simulink model "TWAICE_Cell_Model_Farasis_P75_75Ah_v8_1_3"  (R2017b)
settings: Solver=ode3  StartTime=t_start  StopTime=t_end  FixedStep=Ts  RelTol=1e-3
InitFcn:
  | m = Simulink.Mask.get(strcat(model,'/Virtual Battery Tester'));
  | cycler_selection_sel = m.getParameter('cycler_selection');
  | ts_data_repeat_tickbox_sel = m.getParameter('ts_data_repeat_tickbox');
  | if strcmp(cycler_selection_sel.Value, 'Cycle Generator')
  |      t_end = 60*60*24*365*8;
  | elseif strcmp(cycler_selection_sel.Value, 'Timeseries Data')
  |      if strcmp(ts_data_repeat_tickbox_sel.Value, 'off')
  |           t_end = Data.Time(end);
  |      elseif strcmp(ts_data_repeat_tickbox_sel.Value, 'on')
  |            t_end = 60*60*24*365*8;
  |      end
  | end
StartFcn:
  | m = Simulink.Mask.get(strcat(model,'/Virtual Battery Tester'));
  | cycler_selection_sel = m.getParameter('cycler_selection');
  | ts_data_repeat_tickbox_sel = m.getParameter('ts_data_repeat_tickbox');
  | if strcmp(cycler_selection_sel.Value, 'Cycle Generator')
  |      t_end = 60*60*24*365*8;
  | elseif strcmp(cycler_selection_sel.Value, 'Timeseries Data')
  |      if strcmp(ts_data_repeat_tickbox_sel.Value, 'off')
  |           t_end = Data.Time(end);
  |      elseif strcmp(ts_data_repeat_tickbox_sel.Value, 'on')
  |            t_end = 60*60*24*365*8;
  |      end
  | end
model workspace (MAT data in the model file):
  SOC_init = 1
values from neighbouring files (symbols this model uses):
  act = 1    [RunMe_TWAICE_Cell_Model_Farasis_P75_75Ah_v8_1_3.m]
  I_chlim = []    [RunMe_TWAICE_Cell_Model_Farasis_P75_75Ah_v8_1_3.m]
  I_dislim = []    [RunMe_TWAICE_Cell_Model_Farasis_P75_75Ah_v8_1_3.m]
  lic_no = fin_convert(Prod_lic)    [RunMe_TWAICE_Cell_Model_Farasis_P75_75Ah_v8_1_3.m]
  model = 'TWAICE_Cell_Model_Farasis_P75_75Ah_v8_1_3'    [RunMe_TWAICE_Cell_Model_Farasis_P75_75Ah_v8_1_3.m]
  soc_chlim = chargelim.Var2(inx_soc:end)'    [RunMe_TWAICE_Cell_Model_Farasis_P75_75Ah_v8_1_3.m]
  soc_dislim = dischargelim.Var2(inx_soc:end)'    [RunMe_TWAICE_Cell_Model_Farasis_P75_75Ah_v8_1_3.m]
  T_chlim = []    [RunMe_TWAICE_Cell_Model_Farasis_P75_75Ah_v8_1_3.m]
  T_dislim = []    [RunMe_TWAICE_Cell_Model_Farasis_P75_75Ah_v8_1_3.m]
  Ts = 1    [RunMe_TWAICE_Cell_Model_Farasis_P75_75Ah_v8_1_3.m]
undefined symbols (not defined in the file or in its folder): Data, T_init
libraries: simulink x3
(part 2 of 2)

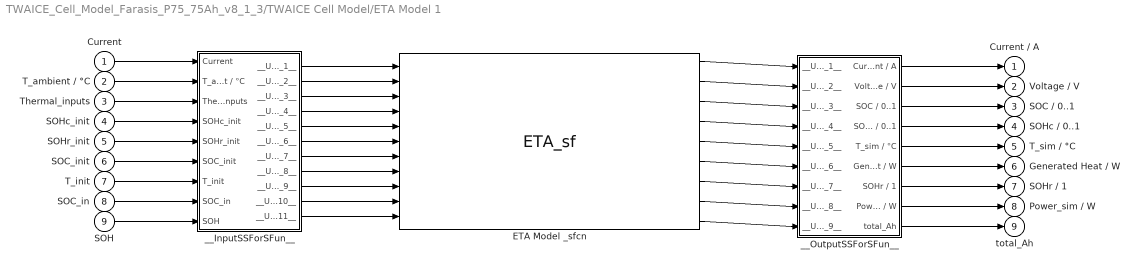
== system TWAICE_Cell_Model_Farasis_P75_75Ah_v8_1_3/TWAICE Cell Model/ETA Model 1 ==
  "Current " : Inport  OutDataTypeStr=double  PortDimensions=1
  T_ambient / °C : Inport  Port=2  OutDataTypeStr=double  PortDimensions=1
  Thermal_inputs : Inport  Port=3
  SOHc_init : Inport  Port=4
  SOHr_init : Inport  Port=5
  SOC_init : Inport  Port=6
  T_init : Inport  Port=7
  SOC_in : Inport  Port=8
  SOH : Inport  Port=9
  ETA Model _sfcn : S-Function  FunctionName=ETA_sf  Parameters=sfcnParam1, sfcnParam2, sfcnParam3  SFunctionModules=""  SFunctionDeploymentMode=off  EnableBusSupport=off  SFcnStateName=DWORK0  mask{rtw_sf_name=ETA_sf, showVar=off, sfcnParam1=sfcnParam1, sfcnParam2=sfcnParam2, sfcnParam3=sfcnParam3}
      mask prompts: rtw_sf_name "Simulink:masks:GenSFuncName_MP"; showVar "Simulink:masks:GenSFuncShowModuleList_MP"; sfcnParam1 "Ts:"; sfcnParam2 "act:"; sfcnParam3 "lic_no:"
      mask help: Simulink:masks:GenSFuncDesc_MD
      mask init:
      | displist = '';
      | if ~strcmp(get_param(gcb, 'FunctionName'), rtw_sf_name);
      |   set_param(gcb, 'FunctionName', rtw_sf_name);
      | end
      | % Check if we are generating code
      | rtw_mode = false;
      | if strcmpi(get_param(bdroot(gcb),'SimulationStatus'),'Initializing')
      | 	rtw_mode = strcmpi(get_param(bdroot(gcb),'BuildingRTWCode'),'on') && ...
      | 		~strcmpi(get_param(bdroot(gcb),'TargetStyle'),'SimulationTarget');
      | end
      | if showVar || rtw_mode
      | 	if exist('rtwsfunc') == 2 | exist('rtwsfunc') == 6
      | 		tmplist = rtwsfunc(rtw_sf_name,gcb);
      | 		tmplist = DAStudio.message('Simulink:masks:GenSFuncListOfModules_IC', tmplist);
      | 	elseif showVar
      | 		tmplist1 = DAStudio.message('Simulink:masks:GenSFuncListOfModules_IC', '');
      |         tmplist2 = DAStudio.message('Simulink:masks:GenSFuncNotLicensed_IC');
      |         tmplist = [tmplist1 tmplist2];
      |  	end
      | end
      | if showVar
      |   displist = tmplist;
      | end
      settings: SFcnIsStateOwnerBlock=on
      settings: CopyFcn=|
      | if ~strcmp(get_param(gcb,'Linkstatus'),'none') && ...
      | ~strcmp(get_param(gcb,'Linkstatus'),'implicit')
      |   set_param(gcb,'LinkStatus','none');
      | end
      mask Help: eval('feval(''rtwprivate'',''rtwhelpview'',''rtw_sfcn_block'')');
      mask Display:
      | port_label('input',1,'Current ');
      | port_label('input',2,'T_ambient / °C');
      | port_label('input',3,'htc_in');
      | port_label('input',4,'Pcool_in');
      | port_label('input',5,'SOHc_init');
      | port_label('input',6,'SOHr_init');
      | port_label('input',7,'SOC_init');
      | port_label('input',8,'T_init');
      | port_label('input',9,'SOC_in');
      | port_label('input',10,'SOHc');
      | port_label('input',11,'SOHr');
      | port_label('output',1,'Current / A');
      | port_label('output',2,'Voltage / V');
      | port_label('output',3,'SOC / 0..1');
      | port_label('output',4,'SOHc / 0..1');
      | port_label('output',5,'T_sim / °C');
      | port_label('output',6,'Generated Heat / W');
      | port_label('output',7,'SOHr / 1');
      | port_label('output',8,'Power_sim / W');
      | port_label('output',9,'total_Ah');
  __InputSSForSFun__ : Subsystem
  __OutputSSForSFun__ : Subsystem
  Current / A : Outport  OutDataTypeStr=double  PortDimensions=1  VectorParamsAs1DForOutWhenUnconnected=on
  Voltage / V : Outport  Port=2  OutDataTypeStr=double  PortDimensions=1  VectorParamsAs1DForOutWhenUnconnected=on
  SOC / 0..1 : Outport  Port=3  OutDataTypeStr=double  PortDimensions=1  VectorParamsAs1DForOutWhenUnconnected=on
  SOHc / 0..1 : Outport  Port=4  OutDataTypeStr=double  PortDimensions=1  VectorParamsAs1DForOutWhenUnconnected=on
  T_sim / °C : Outport  Port=5  OutDataTypeStr=double  PortDimensions=1  VectorParamsAs1DForOutWhenUnconnected=on
  Generated Heat / W : Outport  Port=6  OutDataTypeStr=double  PortDimensions=1  VectorParamsAs1DForOutWhenUnconnected=on
  SOHr / 1 : Outport  Port=7  OutDataTypeStr=double  PortDimensions=1  VectorParamsAs1DForOutWhenUnconnected=on
  Power_sim / W : Outport  Port=8  OutDataTypeStr=double  PortDimensions=1  VectorParamsAs1DForOutWhenUnconnected=on
  total_Ah : Outport  Port=9  VectorParamsAs1DForOutWhenUnconnected=on
  wires:
  "Current "/1 -> __InputSSForSFun__/1("Current ")
  T_ambient / °C/1 -> __InputSSForSFun__/2(T_ambient / °C)
  Thermal_inputs/1 -> __InputSSForSFun__/3(Thermal_inputs)
  SOHc_init/1 -> __InputSSForSFun__/4(SOHc_init)
  SOHr_init/1 -> __InputSSForSFun__/5(SOHr_init)
  SOC_init/1 -> __InputSSForSFun__/6(SOC_init)
  T_init/1 -> __InputSSForSFun__/7(T_init)
  SOC_in/1 -> __InputSSForSFun__/8(SOC_in)
  SOH/1 -> __InputSSForSFun__/9(SOH)
  __InputSSForSFun__/1(__UniqueOutportName__1__) -> ETA Model _sfcn/1
  __InputSSForSFun__/2(__UniqueOutportName__2__) -> ETA Model _sfcn/2
  __InputSSForSFun__/3(__UniqueOutportName__3__) -> ETA Model _sfcn/3
  __InputSSForSFun__/4(__UniqueOutportName__4__) -> ETA Model _sfcn/4
  __InputSSForSFun__/5(__UniqueOutportName__5__) -> ETA Model _sfcn/5
  __InputSSForSFun__/6(__UniqueOutportName__6__) -> ETA Model _sfcn/6
  __InputSSForSFun__/7(__UniqueOutportName__7__) -> ETA Model _sfcn/7
  __InputSSForSFun__/8(__UniqueOutportName__8__) -> ETA Model _sfcn/8
  __InputSSForSFun__/9(__UniqueOutportName__9__) -> ETA Model _sfcn/9
  __InputSSForSFun__/10(__UniqueOutportName__10__) -> ETA Model _sfcn/10
  __InputSSForSFun__/11(__UniqueOutportName__11__) -> ETA Model _sfcn/11
  ETA Model _sfcn/1 -> __OutputSSForSFun__/1(__UniqueInportName__1__)
  ETA Model _sfcn/2 -> __OutputSSForSFun__/2(__UniqueInportName__2__)
  ETA Model _sfcn/3 -> __OutputSSForSFun__/3(__UniqueInportName__3__)
  ETA Model _sfcn/4 -> __OutputSSForSFun__/4(__UniqueInportName__4__)
  ETA Model _sfcn/5 -> __OutputSSForSFun__/5(__UniqueInportName__5__)
  ETA Model _sfcn/6 -> __OutputSSForSFun__/6(__UniqueInportName__6__)
  ETA Model _sfcn/7 -> __OutputSSForSFun__/7(__UniqueInportName__7__)
  ETA Model _sfcn/8 -> __OutputSSForSFun__/8(__UniqueInportName__8__)
  ETA Model _sfcn/9 -> __OutputSSForSFun__/9(__UniqueInportName__9__)
  __OutputSSForSFun__/1(Current / A) -> Current / A/1
  __OutputSSForSFun__/2(Voltage / V) -> Voltage / V/1
  __OutputSSForSFun__/3(SOC / 0..1) -> SOC / 0..1/1
  __OutputSSForSFun__/4(SOHc / 0..1) -> SOHc / 0..1/1
  __OutputSSForSFun__/5(T_sim / °C) -> T_sim / °C/1
  __OutputSSForSFun__/6(Generated Heat / W) -> Generated Heat / W/1
  __OutputSSForSFun__/7(SOHr / 1) -> SOHr / 1/1
  __OutputSSForSFun__/8(Power_sim / W) -> Power_sim / W/1
  __OutputSSForSFun__/9(total_Ah) -> total_Ah/1

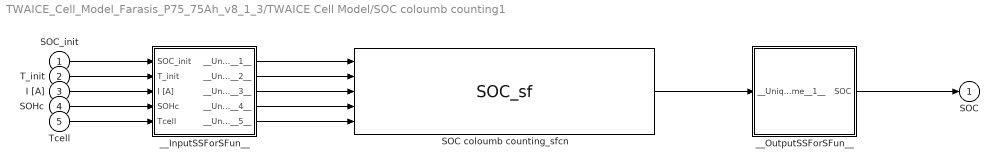
== system TWAICE_Cell_Model_Farasis_P75_75Ah_v8_1_3/TWAICE Cell Model/SOC coloumb counting1 ==
  SOC_init : Inport
  T_init : Inport  Port=2
  I [A] : Inport  Port=3
  SOHc : Inport  Port=4
  Tcell : Inport  Port=5
  SOC coloumb counting_sfcn : S-Function  FunctionName=SOC_sf  Parameters=sfcnParam1  SFunctionModules=""  SFunctionDeploymentMode=off  EnableBusSupport=off  SFcnStateName=DWORK0  mask{rtw_sf_name=SOC_sf, showVar=off, sfcnParam1=sfcnParam1}
      mask prompts: rtw_sf_name "Simulink:masks:GenSFuncName_MP"; showVar "Simulink:masks:GenSFuncShowModuleList_MP"; sfcnParam1 "Ts:"
      mask help: Simulink:masks:GenSFuncDesc_MD
      mask init: same as TWAICE_Cell_Model_Farasis_P75_75Ah_v8_1_3/TWAICE Cell Model/ETA Model 1/ETA Model _sfcn
      settings: SFcnIsStateOwnerBlock=on
      settings: CopyFcn=|
      | if ~strcmp(get_param(gcb,'Linkstatus'),'none') && ...
      | ~strcmp(get_param(gcb,'Linkstatus'),'implicit')
      |   set_param(gcb,'LinkStatus','none');
      | end
      mask Help: eval('feval(''rtwprivate'',''rtwhelpview'',''rtw_sfcn_block'')');
      mask Display:
      | port_label('input',1,'SOC_init');
      | port_label('input',2,'T_init');
      | port_label('input',3,'I [A]');
      | port_label('input',4,'SOHc');
      | port_label('input',5,'Tcell');
      | port_label('output',1,'SOC');
  __InputSSForSFun__ : Subsystem
  __OutputSSForSFun__ : Subsystem
  SOC : Outport
  wires:
  SOC_init/1 -> __InputSSForSFun__/1(SOC_init)
  T_init/1 -> __InputSSForSFun__/2(T_init)
  I [A]/1 -> __InputSSForSFun__/3(I [A])
  SOHc/1 -> __InputSSForSFun__/4(SOHc)
  Tcell/1 -> __InputSSForSFun__/5(Tcell)
  __InputSSForSFun__/1(__UniqueOutportName__1__) -> SOC coloumb counting_sfcn/1
  __InputSSForSFun__/2(__UniqueOutportName__2__) -> SOC coloumb counting_sfcn/2
  __InputSSForSFun__/3(__UniqueOutportName__3__) -> SOC coloumb counting_sfcn/3
  __InputSSForSFun__/4(__UniqueOutportName__4__) -> SOC coloumb counting_sfcn/4
  __InputSSForSFun__/5(__UniqueOutportName__5__) -> SOC coloumb counting_sfcn/5
  SOC coloumb counting_sfcn/1 -> __OutputSSForSFun__/1(__UniqueInportName__1__)
  __OutputSSForSFun__/1(SOC) -> SOC/1

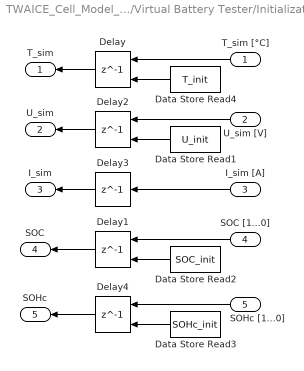
== system TWAICE_Cell_Model_Farasis_P75_75Ah_v8_1_3/Virtual Battery Tester/Initialization ==
  T_sim [°C] : Inport
  U_sim [V] : Inport  Port=2
  I_sim [A] : Inport  Port=3
  SOC [1...0] : Inport  Port=4
  SOHc [1...0] : Inport  Port=5
  Data Store Read1 : DataStoreRead  DataStoreName=U_init
  Data Store Read2 : DataStoreRead  DataStoreName=SOC_init
  Data Store Read3 : DataStoreRead  DataStoreName=SOHc_init
  Data Store Read4 : DataStoreRead  DataStoreName=T_init
  Delay : Delay  DelayLength=1  InitialConditionSource=Input port  InitialCondition=T_init
      settings: InputPortMap=u0,p4
  Delay1 : Delay  DelayLength=1  InitialConditionSource=Input port  InitialCondition=SOC_init
      settings: InputPortMap=u0,p4
  Delay2 : Delay  DelayLength=1  InitialConditionSource=Input port  InitialCondition=3.6
      settings: InputPortMap=u0,p4
  Delay3 : Delay  DelayLength=1  InitialCondition=0
  Delay4 : Delay  DelayLength=1  InitialConditionSource=Input port  InitialCondition=SOC_init
      settings: InputPortMap=u0,p4
  T_sim : Outport  VectorParamsAs1DForOutWhenUnconnected=on
  U_sim : Outport  Port=2  VectorParamsAs1DForOutWhenUnconnected=on
  I_sim : Outport  Port=3  VectorParamsAs1DForOutWhenUnconnected=on
  SOC : Outport  Port=4  VectorParamsAs1DForOutWhenUnconnected=on
  SOHc : Outport  Port=5  VectorParamsAs1DForOutWhenUnconnected=on
  wires:
  T_sim [°C]/1 -> Delay/1
  Delay1/1 -> SOC/1
  Delay2/1 -> U_sim/1
  SOC [1...0]/1 -> Delay1/1
  Delay/1 -> T_sim/1
  I_sim [A]/1 -> Delay3/1
  Delay3/1 -> I_sim/1
  SOHc [1...0]/1 -> Delay4/1
  U_sim [V]/1 -> Delay2/1
  Data Store Read2/1 -> Delay1/2
  Delay4/1 -> SOHc/1
  Data Store Read3/1 -> Delay4/2
  Data Store Read4/1 -> Delay/2
  Data Store Read1/1 -> Delay2/2

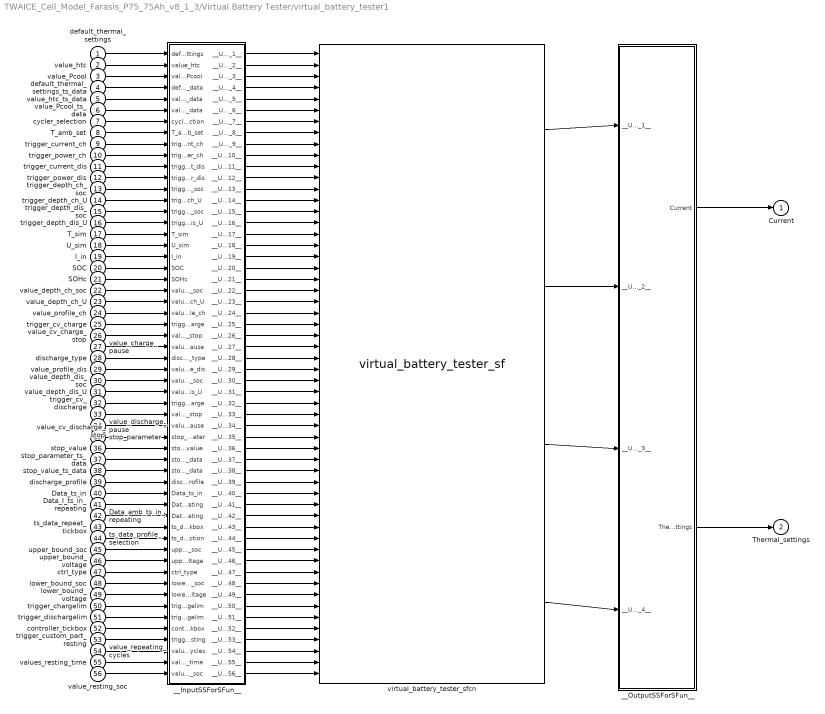
== system TWAICE_Cell_Model_Farasis_P75_75Ah_v8_1_3/Virtual Battery Tester/virtual_battery_tester1 ==
  default_thermal_settings : Inport
  value_htc : Inport  Port=2
  value_Pcool : Inport  Port=3
  default_thermal_settings_ts_data : Inport  Port=4
  value_htc_ts_data : Inport  Port=5
  value_Pcool_ts_data : Inport  Port=6
  cycler_selection : Inport  Port=7
  T_amb_set : Inport  Port=8
  trigger_current_ch : Inport  Port=9
  trigger_power_ch : Inport  Port=10
  trigger_current_dis : Inport  Port=11
  trigger_power_dis : Inport  Port=12
  trigger_depth_ch_soc : Inport  Port=13
  trigger_depth_ch_U : Inport  Port=14
  trigger_depth_dis_soc : Inport  Port=15
  trigger_depth_dis_U : Inport  Port=16
  T_sim : Inport  Port=17
  U_sim : Inport  Port=18
  I_in : Inport  Port=19
  SOC : Inport  Port=20
  SOHc : Inport  Port=21
  value_depth_ch_soc : Inport  Port=22
  value_depth_ch_U : Inport  Port=23
  value_profile_ch : Inport  Port=24
  trigger_cv_charge : Inport  Port=25
  value_cv_charge_stop : Inport  Port=26
  value_charge_pause : Inport  Port=27
  discharge_type : Inport  Port=28
  value_profile_dis : Inport  Port=29
  value_depth_dis_soc : Inport  Port=30
  value_depth_dis_U : Inport  Port=31
  trigger_cv_discharge : Inport  Port=32
  value_cv_discharge_stop : Inport  Port=33
  value_discharge_pause : Inport  Port=34
  stop_parameter : Inport  Port=35
  stop_value : Inport  Port=36
  stop_parameter_ts_data : Inport  Port=37
  stop_value_ts_data : Inport  Port=38
  discharge_profile : Inport  Port=39
  Data_ts_in : Inport  Port=40
  Data_I_ts_in_repeating : Inport  Port=41
  Data_amb_ts_in_repeating : Inport  Port=42
  ts_data_repeat_tickbox : Inport  Port=43
  ts_data_profile_selection : Inport  Port=44
  upper_bound_soc : Inport  Port=45
  upper_bound_voltage : Inport  Port=46
  ctrl_type : Inport  Port=47
  lower_bound_soc : Inport  Port=48
  lower_bound_voltage : Inport  Port=49
  trigger_chargelim : Inport  Port=50
  trigger_dischargelim : Inport  Port=51
  controller_tickbox : Inport  Port=52
  trigger_custom_part_resting : Inport  Port=53
  value_repeating_cycles : Inport  Port=54
  values_resting_time : Inport  Port=55
  value_resting_soc : Inport  Port=56
  __InputSSForSFun__ : Subsystem
  __OutputSSForSFun__ : Subsystem
  virtual_battery_tester_sfcn : S-Function  FunctionName=virtual_battery_tester_sf  Parameters=sfcnParam1, sfcnParam2, sfcnParam3, sfcnParam4, sfcnParam5, sfcnParam6, sfcnParam7, sfcnParam8  SFunctionModules=""  SFunctionDeploymentMode=off  EnableBusSupport=off  SFcnStateName=DWORK0  mask{rtw_sf_name=virtual_battery_tester_sf, showVar=off, sfcnParam1=sfcnParam1, sfcnParam2=sfcnParam2, sfcnParam3=sfcnParam3, sfcnParam4=sfcnParam4, sfcnParam5=sfcnParam5, sfcnParam6=sfcnParam6, sfcnParam7=sfcnParam7, sfcnParam8=sfcnParam8}
      mask prompts: rtw_sf_name "Simulink:masks:GenSFuncName_MP"; showVar "Simulink:masks:GenSFuncShowModuleList_MP"; sfcnParam1 "I_chlim:"; sfcnParam2 "I_dislim:"; sfcnParam3 "T_chlim:"; sfcnParam4 "T_dislim:"; sfcnParam5 "act:"; sfcnParam6 "lic_no:"; sfcnParam7 "soc_chlim:"; sfcnParam8 "soc_dislim:"
      mask help: Simulink:masks:GenSFuncDesc_MD
      mask init: same as TWAICE_Cell_Model_Farasis_P75_75Ah_v8_1_3/TWAICE Cell Model/ETA Model 1/ETA Model _sfcn
      settings: SFcnIsStateOwnerBlock=on
      settings: CopyFcn=|
      | if ~strcmp(get_param(gcb,'Linkstatus'),'none') && ...
      | ~strcmp(get_param(gcb,'Linkstatus'),'implicit')
      |   set_param(gcb,'LinkStatus','none');
      | end
      mask Help: eval('feval(''rtwprivate'',''rtwhelpview'',''rtw_sfcn_block'')');
      mask Display:
      | port_label('input',1,'default_thermal_settings');
      | port_label('input',2,'value_htc');
      | port_label('input',3,'value_Pcool');
      | port_label('input',4,'default_thermal_settings_ts_data');
      | port_label('input',5,'value_htc_ts_data');
      | port_label('input',6,'value_Pcool_ts_data');
      | port_label('input',7,'cycler_selection');
      | port_label('input',8,'T_amb_set');
      | port_label('input',9,'trigger_current_ch');
      | port_label('input',10,'trigger_power_ch');
      | port_label('input',11,'trigger_current_dis');
      | port_label('input',12,'trigger_power_dis');
      | port_label('input',13,'trigger_depth_ch_soc');
      | port_label('input',14,'trigger_depth_ch_U');
      | port_label('input',15,'trigger_depth_dis_soc');
      | port_label('input',16,'trigger_depth_dis_U');
      | port_label('input',17,'T_sim');
      | port_label('input',18,'U_sim');
      | port_label('input',19,'I_in');
      | port_label('input',20,'SOC');
      | port_label('input',21,'SOHc');
      | port_label('input',22,'value_depth_ch_soc');
      | port_label('input',23,'value_depth_ch_U');
      | port_label('input',24,'value_profile_ch');
      | port_label('input',25,'trigger_cv_charge');
      | port_label('input',26,'value_cv_charge_stop');
      | port_label('input',27,'value_charge_pause');
      | port_label('input',28,'discharge_type');
      | port_label('input',29,'value_profile_dis');
      | port_label('input',30,'value_depth_dis_soc');
      | port_label('input',31,'value_depth_dis_U');
      | port_label('input',32,'trigger_cv_discharge');
      | port_label('input',33,'value_cv_discharge_stop');
      | port_label('input',34,'value_discharge_pause');
      | port_label('input',35,'stop_parameter');
      | port_label('input',36,'stop_value');
      | port_label('input',37,'stop_parameter_ts_data');
      | port_label('input',38,'stop_value_ts_data');
      | port_label('input',39,'discharge_profile');
      | port_label('input',40,'Data_ts_in');
      | port_label('input',41,'Data_I_ts_in_repeating');
      | port_label('input',42,'Data_amb_ts_in_repeating');
      | port_label('input',43,'ts_data_repeat_tickbox');
      | port_label('input',44,'ts_data_profile_selection');
      | port_label('input',45,'upper_bound_soc');
      | port_label('input',46,'upper_bound_voltage');
      | port_label('input',47,'ctrl_type');
      | port_label('input',48,'lower_bound_soc');
      | port_label('input',49,'lower_bound_voltage');
      | port_label('input',50,'trigger_chargelim');
      | port_label('input',51,'trigger_dischargelim');
      | port_label('input',52,'controller_tickbox');
      | port_label('input',53,'trigger_custom_part_resting');
      | port_label('input',54,'value_repeating_cycles');
      | port_label('input',55,'values_resting_time');
      | port_label('input',56,'value_resting_soc');
      | port_label('output',1,'Current');
      | port_label('output',2,'T_amb');
      | port_label('output',3,'htc_in');
      | port_label('output',4,'Pcool_in');
  Current : Outport  VectorParamsAs1DForOutWhenUnconnected=on
  Thermal_settings : Outport  Port=2  VectorParamsAs1DForOutWhenUnconnected=on
  wires:
  default_thermal_settings/1 -> __InputSSForSFun__/1(default_thermal_settings)
  value_htc/1 -> __InputSSForSFun__/2(value_htc)
  value_Pcool/1 -> __InputSSForSFun__/3(value_Pcool)
  default_thermal_settings_ts_data/1 -> __InputSSForSFun__/4(default_thermal_settings_ts_data)
  value_htc_ts_data/1 -> __InputSSForSFun__/5(value_htc_ts_data)
  value_Pcool_ts_data/1 -> __InputSSForSFun__/6(value_Pcool_ts_data)
  cycler_selection/1 -> __InputSSForSFun__/7(cycler_selection)
  T_amb_set/1 -> __InputSSForSFun__/8(T_amb_set)
  trigger_current_ch/1 -> __InputSSForSFun__/9(trigger_current_ch)
  trigger_power_ch/1 -> __InputSSForSFun__/10(trigger_power_ch)
  trigger_current_dis/1 -> __InputSSForSFun__/11(trigger_current_dis)
  trigger_power_dis/1 -> __InputSSForSFun__/12(trigger_power_dis)
  trigger_depth_ch_soc/1 -> __InputSSForSFun__/13(trigger_depth_ch_soc)
  trigger_depth_ch_U/1 -> __InputSSForSFun__/14(trigger_depth_ch_U)
  trigger_depth_dis_soc/1 -> __InputSSForSFun__/15(trigger_depth_dis_soc)
  trigger_depth_dis_U/1 -> __InputSSForSFun__/16(trigger_depth_dis_U)
  T_sim/1 -> __InputSSForSFun__/17(T_sim)
  U_sim/1 -> __InputSSForSFun__/18(U_sim)
  I_in/1 -> __InputSSForSFun__/19(I_in)
  SOC/1 -> __InputSSForSFun__/20(SOC)
  SOHc/1 -> __InputSSForSFun__/21(SOHc)
  value_depth_ch_soc/1 -> __InputSSForSFun__/22(value_depth_ch_soc)
  value_depth_ch_U/1 -> __InputSSForSFun__/23(value_depth_ch_U)
  value_profile_ch/1 -> __InputSSForSFun__/24(value_profile_ch)
  trigger_cv_charge/1 -> __InputSSForSFun__/25(trigger_cv_charge)
  value_cv_charge_stop/1 -> __InputSSForSFun__/26(value_cv_charge_stop)
  value_charge_pause/1 -> __InputSSForSFun__/27(value_charge_pause)
  discharge_type/1 -> __InputSSForSFun__/28(discharge_type)
  value_profile_dis/1 -> __InputSSForSFun__/29(value_profile_dis)
  value_depth_dis_soc/1 -> __InputSSForSFun__/30(value_depth_dis_soc)
  value_depth_dis_U/1 -> __InputSSForSFun__/31(value_depth_dis_U)
  trigger_cv_discharge/1 -> __InputSSForSFun__/32(trigger_cv_discharge)
  value_cv_discharge_stop/1 -> __InputSSForSFun__/33(value_cv_discharge_stop)
  value_discharge_pause/1 -> __InputSSForSFun__/34(value_discharge_pause)
  stop_parameter/1 -> __InputSSForSFun__/35(stop_parameter)
  stop_value/1 -> __InputSSForSFun__/36(stop_value)
  stop_parameter_ts_data/1 -> __InputSSForSFun__/37(stop_parameter_ts_data)
  stop_value_ts_data/1 -> __InputSSForSFun__/38(stop_value_ts_data)
  discharge_profile/1 -> __InputSSForSFun__/39(discharge_profile)
  Data_ts_in/1 -> __InputSSForSFun__/40(Data_ts_in)
  Data_I_ts_in_repeating/1 -> __InputSSForSFun__/41(Data_I_ts_in_repeating)
  Data_amb_ts_in_repeating/1 -> __InputSSForSFun__/42(Data_amb_ts_in_repeating)
  ts_data_repeat_tickbox/1 -> __InputSSForSFun__/43(ts_data_repeat_tickbox)
  ts_data_profile_selection/1 -> __InputSSForSFun__/44(ts_data_profile_selection)
  upper_bound_soc/1 -> __InputSSForSFun__/45(upper_bound_soc)
  upper_bound_voltage/1 -> __InputSSForSFun__/46(upper_bound_voltage)
  ctrl_type/1 -> __InputSSForSFun__/47(ctrl_type)
  lower_bound_soc/1 -> __InputSSForSFun__/48(lower_bound_soc)
  lower_bound_voltage/1 -> __InputSSForSFun__/49(lower_bound_voltage)
  trigger_chargelim/1 -> __InputSSForSFun__/50(trigger_chargelim)
  trigger_dischargelim/1 -> __InputSSForSFun__/51(trigger_dischargelim)
  controller_tickbox/1 -> __InputSSForSFun__/52(controller_tickbox)
  trigger_custom_part_resting/1 -> __InputSSForSFun__/53(trigger_custom_part_resting)
  value_repeating_cycles/1 -> __InputSSForSFun__/54(value_repeating_cycles)
  values_resting_time/1 -> __InputSSForSFun__/55(values_resting_time)
  value_resting_soc/1 -> __InputSSForSFun__/56(value_resting_soc)
  __InputSSForSFun__/1(__UniqueOutportName__1__) -> virtual_battery_tester_sfcn/1
  __InputSSForSFun__/2(__UniqueOutportName__2__) -> virtual_battery_tester_sfcn/2
  __InputSSForSFun__/3(__UniqueOutportName__3__) -> virtual_battery_tester_sfcn/3
  __InputSSForSFun__/4(__UniqueOutportName__4__) -> virtual_battery_tester_sfcn/4
  __InputSSForSFun__/5(__UniqueOutportName__5__) -> virtual_battery_tester_sfcn/5
  __InputSSForSFun__/6(__UniqueOutportName__6__) -> virtual_battery_tester_sfcn/6
  __InputSSForSFun__/7(__UniqueOutportName__7__) -> virtual_battery_tester_sfcn/7
  __InputSSForSFun__/8(__UniqueOutportName__8__) -> virtual_battery_tester_sfcn/8
  __InputSSForSFun__/9(__UniqueOutportName__9__) -> virtual_battery_tester_sfcn/9
  __InputSSForSFun__/10(__UniqueOutportName__10__) -> virtual_battery_tester_sfcn/10
  __InputSSForSFun__/11(__UniqueOutportName__11__) -> virtual_battery_tester_sfcn/11
  __InputSSForSFun__/12(__UniqueOutportName__12__) -> virtual_battery_tester_sfcn/12
  __InputSSForSFun__/13(__UniqueOutportName__13__) -> virtual_battery_tester_sfcn/13
  __InputSSForSFun__/14(__UniqueOutportName__14__) -> virtual_battery_tester_sfcn/14
  __InputSSForSFun__/15(__UniqueOutportName__15__) -> virtual_battery_tester_sfcn/15
  __InputSSForSFun__/16(__UniqueOutportName__16__) -> virtual_battery_tester_sfcn/16
  __InputSSForSFun__/17(__UniqueOutportName__17__) -> virtual_battery_tester_sfcn/17
  __InputSSForSFun__/18(__UniqueOutportName__18__) -> virtual_battery_tester_sfcn/18
  __InputSSForSFun__/19(__UniqueOutportName__19__) -> virtual_battery_tester_sfcn/19
  __InputSSForSFun__/20(__UniqueOutportName__20__) -> virtual_battery_tester_sfcn/20
  __InputSSForSFun__/21(__UniqueOutportName__21__) -> virtual_battery_tester_sfcn/21
  __InputSSForSFun__/22(__UniqueOutportName__22__) -> virtual_battery_tester_sfcn/22
  __InputSSForSFun__/23(__UniqueOutportName__23__) -> virtual_battery_tester_sfcn/23
  __InputSSForSFun__/24(__UniqueOutportName__24__) -> virtual_battery_tester_sfcn/24
  __InputSSForSFun__/25(__UniqueOutportName__25__) -> virtual_battery_tester_sfcn/25
  __InputSSForSFun__/26(__UniqueOutportName__26__) -> virtual_battery_tester_sfcn/26
  __InputSSForSFun__/27(__UniqueOutportName__27__) -> virtual_battery_tester_sfcn/27
  __InputSSForSFun__/28(__UniqueOutportName__28__) -> virtual_battery_tester_sfcn/28
  __InputSSForSFun__/29(__UniqueOutportName__29__) -> virtual_battery_tester_sfcn/29
  __InputSSForSFun__/30(__UniqueOutportName__30__) -> virtual_battery_tester_sfcn/30
  __InputSSForSFun__/31(__UniqueOutportName__31__) -> virtual_battery_tester_sfcn/31
  __InputSSForSFun__/32(__UniqueOutportName__32__) -> virtual_battery_tester_sfcn/32
  __InputSSForSFun__/33(__UniqueOutportName__33__) -> virtual_battery_tester_sfcn/33
  __InputSSForSFun__/34(__UniqueOutportName__34__) -> virtual_battery_tester_sfcn/34
  __InputSSForSFun__/35(__UniqueOutportName__35__) -> virtual_battery_tester_sfcn/35
  __InputSSForSFun__/36(__UniqueOutportName__36__) -> virtual_battery_tester_sfcn/36
  __InputSSForSFun__/37(__UniqueOutportName__37__) -> virtual_battery_tester_sfcn/37
  __InputSSForSFun__/38(__UniqueOutportName__38__) -> virtual_battery_tester_sfcn/38
  __InputSSForSFun__/39(__UniqueOutportName__39__) -> virtual_battery_tester_sfcn/39
  __InputSSForSFun__/40(__UniqueOutportName__40__) -> virtual_battery_tester_sfcn/40
  __InputSSForSFun__/41(__UniqueOutportName__41__) -> virtual_battery_tester_sfcn/41
  __InputSSForSFun__/42(__UniqueOutportName__42__) -> virtual_battery_tester_sfcn/42
  __InputSSForSFun__/43(__UniqueOutportName__43__) -> virtual_battery_tester_sfcn/43
  __InputSSForSFun__/44(__UniqueOutportName__44__) -> virtual_battery_tester_sfcn/44
  __InputSSForSFun__/45(__UniqueOutportName__45__) -> virtual_battery_tester_sfcn/45
  __InputSSForSFun__/46(__UniqueOutportName__46__) -> virtual_battery_tester_sfcn/46
  __InputSSForSFun__/47(__UniqueOutportName__47__) -> virtual_battery_tester_sfcn/47
  __InputSSForSFun__/48(__UniqueOutportName__48__) -> virtual_battery_tester_sfcn/48
  __InputSSForSFun__/49(__UniqueOutportName__49__) -> virtual_battery_tester_sfcn/49
  __InputSSForSFun__/50(__UniqueOutportName__50__) -> virtual_battery_tester_sfcn/50
  __InputSSForSFun__/51(__UniqueOutportName__51__) -> virtual_battery_tester_sfcn/51
  __InputSSForSFun__/52(__UniqueOutportName__52__) -> virtual_battery_tester_sfcn/52
  __InputSSForSFun__/53(__UniqueOutportName__53__) -> virtual_battery_tester_sfcn/53
  __InputSSForSFun__/54(__UniqueOutportName__54__) -> virtual_battery_tester_sfcn/54
  __InputSSForSFun__/55(__UniqueOutportName__55__) -> virtual_battery_tester_sfcn/55
  __InputSSForSFun__/56(__UniqueOutportName__56__) -> virtual_battery_tester_sfcn/56
  virtual_battery_tester_sfcn/1 -> __OutputSSForSFun__/1(__UniqueInportName__1__)
  virtual_battery_tester_sfcn/2 -> __OutputSSForSFun__/2(__UniqueInportName__2__)
  virtual_battery_tester_sfcn/3 -> __OutputSSForSFun__/3(__UniqueInportName__3__)
  virtual_battery_tester_sfcn/4 -> __OutputSSForSFun__/4(__UniqueInportName__4__)
  __OutputSSForSFun__/1(Current) -> Current/1
  __OutputSSForSFun__/2(Thermal_settings) -> Thermal_settings/1

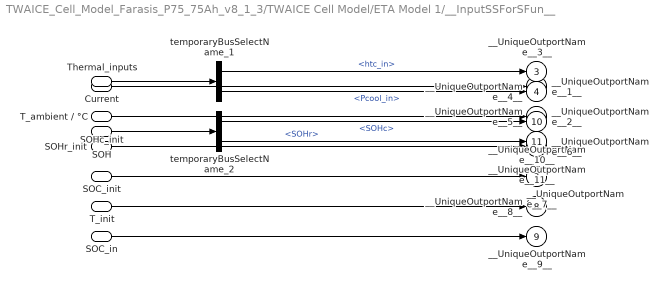
== system TWAICE_Cell_Model_Farasis_P75_75Ah_v8_1_3/TWAICE Cell Model/ETA Model 1/__InputSSForSFun__ ==
  "Current " : Inport  OutDataTypeStr=double  PortDimensions=1
  T_ambient / °C : Inport  Port=2  OutDataTypeStr=double  PortDimensions=1
  Thermal_inputs : Inport  Port=3
  SOHc_init : Inport  Port=4
  SOHr_init : Inport  Port=5
  SOC_init : Inport  Port=6
  T_init : Inport  Port=7
  SOC_in : Inport  Port=8
  SOH : Inport  Port=9
  temporaryBusSelectName_1 : BusSelector  OutputSignals=htc_in,Pcool_in
  temporaryBusSelectName_2 : BusSelector  OutputSignals=SOHc,SOHr
  __UniqueOutportName__1__ : Outport
  __UniqueOutportName__2__ : Outport  Port=2
  __UniqueOutportName__3__ : Outport  Port=3
  __UniqueOutportName__4__ : Outport  Port=4
  __UniqueOutportName__5__ : Outport  Port=5
  __UniqueOutportName__6__ : Outport  Port=6
  __UniqueOutportName__7__ : Outport  Port=7
  __UniqueOutportName__8__ : Outport  Port=8
  __UniqueOutportName__9__ : Outport  Port=9
  __UniqueOutportName__10__ : Outport  Port=10
  __UniqueOutportName__11__ : Outport  Port=11
  wires:
  Thermal_inputs/1 -> temporaryBusSelectName_1/1
  SOH/1 -> temporaryBusSelectName_2/1
  "Current "/1 -> __UniqueOutportName__1__/1
  T_ambient / °C/1 -> __UniqueOutportName__2__/1
  temporaryBusSelectName_1/1 -> __UniqueOutportName__3__/1  "<htc_in>"
  temporaryBusSelectName_1/2 -> __UniqueOutportName__4__/1  "<Pcool_in>"
  SOHc_init/1 -> __UniqueOutportName__5__/1
  SOHr_init/1 -> __UniqueOutportName__6__/1
  SOC_init/1 -> __UniqueOutportName__7__/1
  T_init/1 -> __UniqueOutportName__8__/1
  SOC_in/1 -> __UniqueOutportName__9__/1
  temporaryBusSelectName_2/1 -> __UniqueOutportName__10__/1  "<SOHc>"
  temporaryBusSelectName_2/2 -> __UniqueOutportName__11__/1  "<SOHr>"

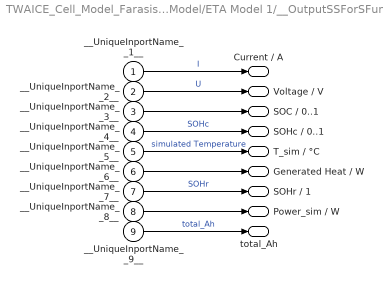
== system TWAICE_Cell_Model_Farasis_P75_75Ah_v8_1_3/TWAICE Cell Model/ETA Model 1/__OutputSSForSFun__ ==
  __UniqueInportName__1__ : Inport
  __UniqueInportName__2__ : Inport  Port=2
  __UniqueInportName__3__ : Inport  Port=3
  __UniqueInportName__4__ : Inport  Port=4
  __UniqueInportName__5__ : Inport  Port=5
  __UniqueInportName__6__ : Inport  Port=6
  __UniqueInportName__7__ : Inport  Port=7
  __UniqueInportName__8__ : Inport  Port=8
  __UniqueInportName__9__ : Inport  Port=9
  Current / A : Outport  OutDataTypeStr=double  PortDimensions=1  VectorParamsAs1DForOutWhenUnconnected=on
  Voltage / V : Outport  Port=2  OutDataTypeStr=double  PortDimensions=1  VectorParamsAs1DForOutWhenUnconnected=on
  SOC / 0..1 : Outport  Port=3  OutDataTypeStr=double  PortDimensions=1  VectorParamsAs1DForOutWhenUnconnected=on
  SOHc / 0..1 : Outport  Port=4  OutDataTypeStr=double  PortDimensions=1  VectorParamsAs1DForOutWhenUnconnected=on
  T_sim / °C : Outport  Port=5  OutDataTypeStr=double  PortDimensions=1  VectorParamsAs1DForOutWhenUnconnected=on
  Generated Heat / W : Outport  Port=6  OutDataTypeStr=double  PortDimensions=1  VectorParamsAs1DForOutWhenUnconnected=on
  SOHr / 1 : Outport  Port=7  OutDataTypeStr=double  PortDimensions=1  VectorParamsAs1DForOutWhenUnconnected=on
  Power_sim / W : Outport  Port=8  OutDataTypeStr=double  PortDimensions=1  VectorParamsAs1DForOutWhenUnconnected=on
  total_Ah : Outport  Port=9  VectorParamsAs1DForOutWhenUnconnected=on
  wires:
  __UniqueInportName__1__/1 -> Current / A/1  "I"
  __UniqueInportName__2__/1 -> Voltage / V/1  "U"
  __UniqueInportName__3__/1 -> SOC / 0..1/1
  __UniqueInportName__4__/1 -> SOHc / 0..1/1  "SOHc"
  __UniqueInportName__5__/1 -> T_sim / °C/1  "simulated Temperature"
  __UniqueInportName__6__/1 -> Generated Heat / W/1
  __UniqueInportName__7__/1 -> SOHr / 1/1  "SOHr"
  __UniqueInportName__8__/1 -> Power_sim / W/1
  __UniqueInportName__9__/1 -> total_Ah/1  "total_Ah"

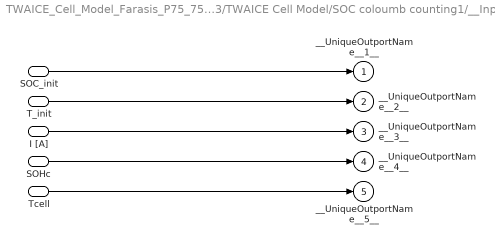
== system TWAICE_Cell_Model_Farasis_P75_75Ah_v8_1_3/TWAICE Cell Model/SOC coloumb counting1/__InputSSForSFun__ ==
  SOC_init : Inport
  T_init : Inport  Port=2
  I [A] : Inport  Port=3
  SOHc : Inport  Port=4
  Tcell : Inport  Port=5
  __UniqueOutportName__1__ : Outport
  __UniqueOutportName__2__ : Outport  Port=2
  __UniqueOutportName__3__ : Outport  Port=3
  __UniqueOutportName__4__ : Outport  Port=4
  __UniqueOutportName__5__ : Outport  Port=5
  wires:
  SOC_init/1 -> __UniqueOutportName__1__/1
  T_init/1 -> __UniqueOutportName__2__/1
  I [A]/1 -> __UniqueOutportName__3__/1
  SOHc/1 -> __UniqueOutportName__4__/1
  Tcell/1 -> __UniqueOutportName__5__/1

== system TWAICE_Cell_Model_Farasis_P75_75Ah_v8_1_3/TWAICE Cell Model/SOC coloumb counting1/__OutputSSForSFun__ ==
  __UniqueInportName__1__ : Inport
  SOC : Outport
  wires:
  __UniqueInportName__1__/1 -> SOC/1

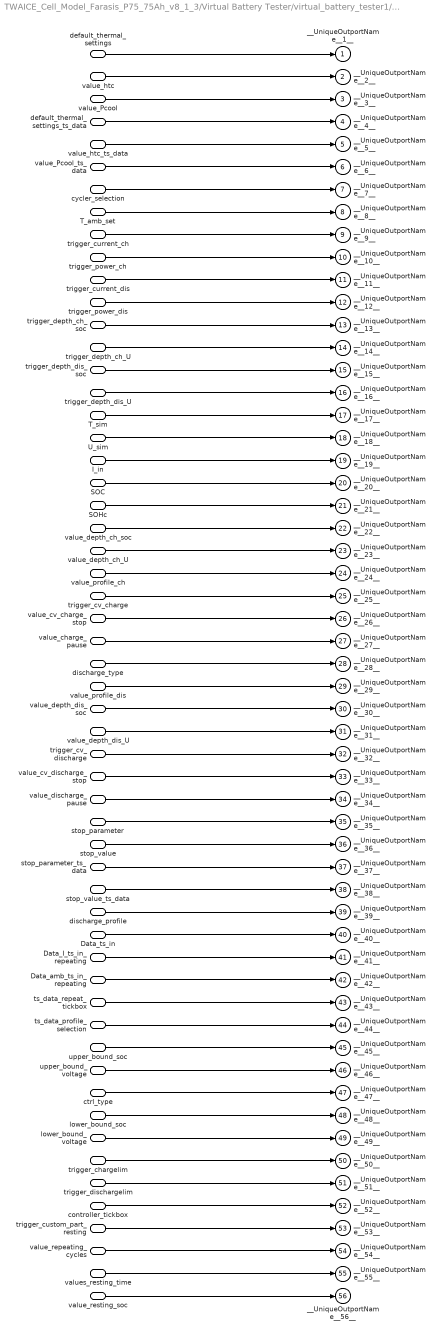
== system TWAICE_Cell_Model_Farasis_P75_75Ah_v8_1_3/Virtual Battery Tester/virtual_battery_tester1/__InputSSForSFun__ ==
  default_thermal_settings : Inport
  value_htc : Inport  Port=2
  value_Pcool : Inport  Port=3
  default_thermal_settings_ts_data : Inport  Port=4
  value_htc_ts_data : Inport  Port=5
  value_Pcool_ts_data : Inport  Port=6
  cycler_selection : Inport  Port=7
  T_amb_set : Inport  Port=8
  trigger_current_ch : Inport  Port=9
  trigger_power_ch : Inport  Port=10
  trigger_current_dis : Inport  Port=11
  trigger_power_dis : Inport  Port=12
  trigger_depth_ch_soc : Inport  Port=13
  trigger_depth_ch_U : Inport  Port=14
  trigger_depth_dis_soc : Inport  Port=15
  trigger_depth_dis_U : Inport  Port=16
  T_sim : Inport  Port=17
  U_sim : Inport  Port=18
  I_in : Inport  Port=19
  SOC : Inport  Port=20
  SOHc : Inport  Port=21
  value_depth_ch_soc : Inport  Port=22
  value_depth_ch_U : Inport  Port=23
  value_profile_ch : Inport  Port=24
  trigger_cv_charge : Inport  Port=25
  value_cv_charge_stop : Inport  Port=26
  value_charge_pause : Inport  Port=27
  discharge_type : Inport  Port=28
  value_profile_dis : Inport  Port=29
  value_depth_dis_soc : Inport  Port=30
  value_depth_dis_U : Inport  Port=31
  trigger_cv_discharge : Inport  Port=32
  value_cv_discharge_stop : Inport  Port=33
  value_discharge_pause : Inport  Port=34
  stop_parameter : Inport  Port=35
  stop_value : Inport  Port=36
  stop_parameter_ts_data : Inport  Port=37
  stop_value_ts_data : Inport  Port=38
  discharge_profile : Inport  Port=39
  Data_ts_in : Inport  Port=40
  Data_I_ts_in_repeating : Inport  Port=41
  Data_amb_ts_in_repeating : Inport  Port=42
  ts_data_repeat_tickbox : Inport  Port=43
  ts_data_profile_selection : Inport  Port=44
  upper_bound_soc : Inport  Port=45
  upper_bound_voltage : Inport  Port=46
  ctrl_type : Inport  Port=47
  lower_bound_soc : Inport  Port=48
  lower_bound_voltage : Inport  Port=49
  trigger_chargelim : Inport  Port=50
  trigger_dischargelim : Inport  Port=51
  controller_tickbox : Inport  Port=52
  trigger_custom_part_resting : Inport  Port=53
  value_repeating_cycles : Inport  Port=54
  values_resting_time : Inport  Port=55
  value_resting_soc : Inport  Port=56
  __UniqueOutportName__1__ : Outport
  __UniqueOutportName__2__ : Outport  Port=2
  __UniqueOutportName__3__ : Outport  Port=3
  __UniqueOutportName__4__ : Outport  Port=4
  __UniqueOutportName__5__ : Outport  Port=5
  __UniqueOutportName__6__ : Outport  Port=6
  __UniqueOutportName__7__ : Outport  Port=7
  __UniqueOutportName__8__ : Outport  Port=8
  __UniqueOutportName__9__ : Outport  Port=9
  __UniqueOutportName__10__ : Outport  Port=10
  __UniqueOutportName__11__ : Outport  Port=11
  __UniqueOutportName__12__ : Outport  Port=12
  __UniqueOutportName__13__ : Outport  Port=13
  __UniqueOutportName__14__ : Outport  Port=14
  __UniqueOutportName__15__ : Outport  Port=15
  __UniqueOutportName__16__ : Outport  Port=16
  __UniqueOutportName__17__ : Outport  Port=17
  __UniqueOutportName__18__ : Outport  Port=18
  __UniqueOutportName__19__ : Outport  Port=19
  __UniqueOutportName__20__ : Outport  Port=20
  __UniqueOutportName__21__ : Outport  Port=21
  __UniqueOutportName__22__ : Outport  Port=22
  __UniqueOutportName__23__ : Outport  Port=23
  __UniqueOutportName__24__ : Outport  Port=24
  __UniqueOutportName__25__ : Outport  Port=25
  __UniqueOutportName__26__ : Outport  Port=26
  __UniqueOutportName__27__ : Outport  Port=27
  __UniqueOutportName__28__ : Outport  Port=28
  __UniqueOutportName__29__ : Outport  Port=29
  __UniqueOutportName__30__ : Outport  Port=30
  __UniqueOutportName__31__ : Outport  Port=31
  __UniqueOutportName__32__ : Outport  Port=32
  __UniqueOutportName__33__ : Outport  Port=33
  __UniqueOutportName__34__ : Outport  Port=34
  __UniqueOutportName__35__ : Outport  Port=35
  __UniqueOutportName__36__ : Outport  Port=36
  __UniqueOutportName__37__ : Outport  Port=37
  __UniqueOutportName__38__ : Outport  Port=38
  __UniqueOutportName__39__ : Outport  Port=39
  __UniqueOutportName__40__ : Outport  Port=40
  __UniqueOutportName__41__ : Outport  Port=41
  __UniqueOutportName__42__ : Outport  Port=42
  __UniqueOutportName__43__ : Outport  Port=43
  __UniqueOutportName__44__ : Outport  Port=44
  __UniqueOutportName__45__ : Outport  Port=45
  __UniqueOutportName__46__ : Outport  Port=46
  __UniqueOutportName__47__ : Outport  Port=47
  __UniqueOutportName__48__ : Outport  Port=48
  __UniqueOutportName__49__ : Outport  Port=49
  __UniqueOutportName__50__ : Outport  Port=50
  __UniqueOutportName__51__ : Outport  Port=51
  __UniqueOutportName__52__ : Outport  Port=52
  __UniqueOutportName__53__ : Outport  Port=53
  __UniqueOutportName__54__ : Outport  Port=54
  __UniqueOutportName__55__ : Outport  Port=55
  __UniqueOutportName__56__ : Outport  Port=56
  wires:
  default_thermal_settings/1 -> __UniqueOutportName__1__/1
  value_htc/1 -> __UniqueOutportName__2__/1
  value_Pcool/1 -> __UniqueOutportName__3__/1
  default_thermal_settings_ts_data/1 -> __UniqueOutportName__4__/1
  value_htc_ts_data/1 -> __UniqueOutportName__5__/1
  value_Pcool_ts_data/1 -> __UniqueOutportName__6__/1
  cycler_selection/1 -> __UniqueOutportName__7__/1
  T_amb_set/1 -> __UniqueOutportName__8__/1
  trigger_current_ch/1 -> __UniqueOutportName__9__/1
  trigger_power_ch/1 -> __UniqueOutportName__10__/1
  trigger_current_dis/1 -> __UniqueOutportName__11__/1
  trigger_power_dis/1 -> __UniqueOutportName__12__/1
  trigger_depth_ch_soc/1 -> __UniqueOutportName__13__/1
  trigger_depth_ch_U/1 -> __UniqueOutportName__14__/1
  trigger_depth_dis_soc/1 -> __UniqueOutportName__15__/1
  trigger_depth_dis_U/1 -> __UniqueOutportName__16__/1
  T_sim/1 -> __UniqueOutportName__17__/1
  U_sim/1 -> __UniqueOutportName__18__/1
  I_in/1 -> __UniqueOutportName__19__/1
  SOC/1 -> __UniqueOutportName__20__/1
  SOHc/1 -> __UniqueOutportName__21__/1
  value_depth_ch_soc/1 -> __UniqueOutportName__22__/1
  value_depth_ch_U/1 -> __UniqueOutportName__23__/1
  value_profile_ch/1 -> __UniqueOutportName__24__/1
  trigger_cv_charge/1 -> __UniqueOutportName__25__/1
  value_cv_charge_stop/1 -> __UniqueOutportName__26__/1
  value_charge_pause/1 -> __UniqueOutportName__27__/1
  discharge_type/1 -> __UniqueOutportName__28__/1
  value_profile_dis/1 -> __UniqueOutportName__29__/1
  value_depth_dis_soc/1 -> __UniqueOutportName__30__/1
  value_depth_dis_U/1 -> __UniqueOutportName__31__/1
  trigger_cv_discharge/1 -> __UniqueOutportName__32__/1
  value_cv_discharge_stop/1 -> __UniqueOutportName__33__/1
  value_discharge_pause/1 -> __UniqueOutportName__34__/1
  stop_parameter/1 -> __UniqueOutportName__35__/1
  stop_value/1 -> __UniqueOutportName__36__/1
  stop_parameter_ts_data/1 -> __UniqueOutportName__37__/1
  stop_value_ts_data/1 -> __UniqueOutportName__38__/1
  discharge_profile/1 -> __UniqueOutportName__39__/1
  Data_ts_in/1 -> __UniqueOutportName__40__/1
  Data_I_ts_in_repeating/1 -> __UniqueOutportName__41__/1
  Data_amb_ts_in_repeating/1 -> __UniqueOutportName__42__/1
  ts_data_repeat_tickbox/1 -> __UniqueOutportName__43__/1
  ts_data_profile_selection/1 -> __UniqueOutportName__44__/1
  upper_bound_soc/1 -> __UniqueOutportName__45__/1
  upper_bound_voltage/1 -> __UniqueOutportName__46__/1
  ctrl_type/1 -> __UniqueOutportName__47__/1
  lower_bound_soc/1 -> __UniqueOutportName__48__/1
  lower_bound_voltage/1 -> __UniqueOutportName__49__/1
  trigger_chargelim/1 -> __UniqueOutportName__50__/1
  trigger_dischargelim/1 -> __UniqueOutportName__51__/1
  controller_tickbox/1 -> __UniqueOutportName__52__/1
  trigger_custom_part_resting/1 -> __UniqueOutportName__53__/1
  value_repeating_cycles/1 -> __UniqueOutportName__54__/1
  values_resting_time/1 -> __UniqueOutportName__55__/1
  value_resting_soc/1 -> __UniqueOutportName__56__/1

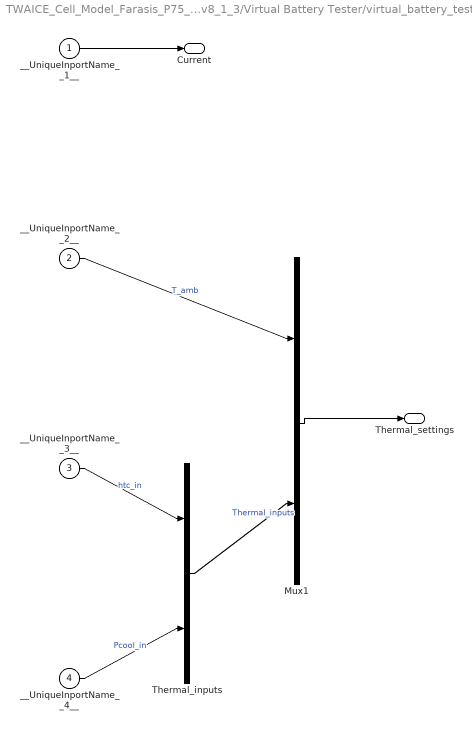
== system TWAICE_Cell_Model_Farasis_P75_75Ah_v8_1_3/Virtual Battery Tester/virtual_battery_tester1/__OutputSSForSFun__ ==
  __UniqueInportName__1__ : Inport
  __UniqueInportName__2__ : Inport  Port=2
  __UniqueInportName__3__ : Inport  Port=3
  __UniqueInportName__4__ : Inport  Port=4
  Mux1 : BusCreator  Inputs=2
  Thermal_inputs : BusCreator  Inputs=2
  Current : Outport  VectorParamsAs1DForOutWhenUnconnected=on
  Thermal_settings : Outport  Port=2  VectorParamsAs1DForOutWhenUnconnected=on
  wires:
  __UniqueInportName__1__/1 -> Current/1
  __UniqueInportName__3__/1 -> Thermal_inputs/1  "htc_in"
  __UniqueInportName__4__/1 -> Thermal_inputs/2  "Pcool_in"
  __UniqueInportName__2__/1 -> Mux1/1  "T_amb"
  Thermal_inputs/1 -> Mux1/2  "Thermal_inputs"
  Mux1/1 -> Thermal_settings/1
